simulink model "hydCircuit"  (R2015a)
settings: Solver=ode23t  StartTime=0.0  StopTime=1  RelTol=1e-3  AbsTol=1e-3
libraries: fl_lib x7, nesl_utility x3
settings Model: Creator=scastro  LastModifiedBy=sseshadr
settings SimscapeCC: SimscapeLogType=all  SimscapeLogDataHistory=10000

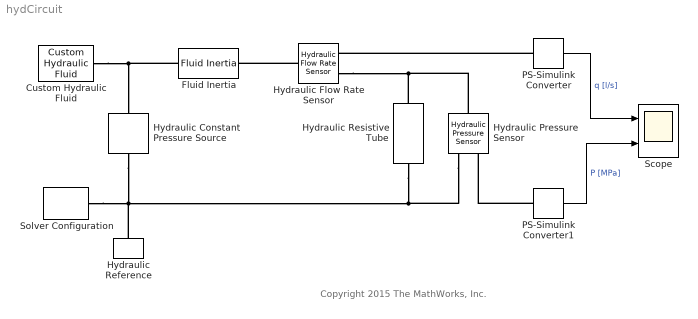
== system hydCircuit ==
  note: Copyright 2015 The MathWorks, Inc.
  Custom Hydraulic Fluid : fl_lib/Hydraulic/Hydraulic Utilities/Custom Hydraulic Fluid  density=850 kg/m^3  viscosity_kin=18e-6 m^2/s  bulk=0.8e9 Pa  alpha=0.005  range_error=2
  Fluid Inertia : fl_lib/Hydraulic/Hydraulic Elements/Fluid Inertia  area=7e-4 m^2  length=1 m  q_specify=off  q_priority=High  q=0.001 m^3/s  p_specify=off  p_priority=High  p=0 Pa
  Hydraulic Pressure Sensor : fl_lib/Hydraulic/Hydraulic Sensors/Hydraulic Pressure Sensor
  Hydraulic Resistive Tube : fl_lib/Hydraulic/Hydraulic Elements/Hydraulic Resistive Tube  cs_type=1  d_in=0.03 m  area=1e-4 m^2  D_h=1.12e-2 m  s_factor=64  length=1 m  length_ad=1 m  roughness=15e-6 m  Re_lam=2000  Re_turb=4000  length_eff=6 m  rel_roughness=0.001  q_specify=off  q_priority=High  q=0.001 m^3/s  p_specify=off  p_priority=High  p=0 Pa
  Hydraulic Constant Pressure Source : fl_lib/Hydraulic/Hydraulic Sources/Hydraulic Constant Pressure Source  commanded_pressure=1 MPa
  Hydraulic Flow Rate Sensor : fl_lib/Hydraulic/Hydraulic Sensors/Hydraulic Flow Rate Sensor
  Hydraulic Reference : fl_lib/Hydraulic/Hydraulic Elements/Hydraulic Reference
  PS-Simulink Converter : nesl_utility/PS-Simulink Converter  PhysicalDomain=network_engine_domain  SubClassName=ps_output  LeftPortType=input  RightPortType=output  PseudoPeriodic=off  Frequencies=[]  Unit=l/s  AffineConversion=off
  PS-Simulink Converter1 : nesl_utility/PS-Simulink Converter  PhysicalDomain=network_engine_domain  SubClassName=ps_output  LeftPortType=input  RightPortType=output  PseudoPeriodic=off  Frequencies=[]  Unit=MPa  AffineConversion=off
  Scope : Scope  NumInputPorts=2
      settings: TimeRange=1  YMin=0~0  YMax=30~1.5
  Solver Configuration : nesl_utility/Solver Configuration  PhysicalDomain=network_engine_domain  SubClassName=solver  LeftPortType=input  RightPortType=generic  Accelerate=off  Tones=[]  Harmonics=[]  SimulateNoise=off  Profile=off  UseLocalSampling=off  EnableSwitchedLinearOptims=on  FrequencyDomain=off  UseCCode=off  RelTol=0.001  AbsTol=1e-06  MinStep=1e-09  ToWorkspace=off  RevertToSquareIcSolve=off  NumHomotopyIterations=100  DoDC=off  ResidualTolerance=1e-09  UseLocalSolver=off  LocalSolverChoice=NE_BACKWARD_EULER_ADVANCER  LocalSolverSampleTime=0.001  DoFixedCost=off  MaxNonlinIter=3  MaxModeIter=2  LinearAlgebra=Sparse  DelaysMemoryBudget=1024  AutomaticFiltering=on  FilteringTimeConstant=0.001
  wires:
  PS-Simulink Converter/1 -> Scope/1  "q [l/s]"
  PS-Simulink Converter1/1 -> Scope/2  "P [MPa]"
  connections:
  Fluid Inertia/LConn1 -- Hydraulic Constant Pressure Source/LConn1 -- Custom Hydraulic Fluid/RConn1
  Hydraulic Flow Rate Sensor/LConn1 -- Fluid Inertia/RConn1
  Hydraulic Flow Rate Sensor/RConn2 -- Hydraulic Resistive Tube/LConn1 -- Hydraulic Pressure Sensor/LConn1
  Hydraulic Constant Pressure Source/RConn1 -- Hydraulic Reference/LConn1 -- Hydraulic Resistive Tube/RConn1 -- Hydraulic Pressure Sensor/RConn1 -- Solver Configuration/RConn1
  PS-Simulink Converter/LConn1 -- Hydraulic Flow Rate Sensor/RConn1
  PS-Simulink Converter1/LConn1 -- Hydraulic Pressure Sensor/RConn2
